simulink model "building_PHPP_v1"  (R2018b)
settings: Solver=ode23s  StartTime=-building.preruntime+8760*3600  StopTime=building.runtime+8760*3600  EnableMultiTasking=on
StartFcn:
  | tic
StopFcn:
  | toc
values from neighbouring files (symbols this model uses):
  A = 7*10*2    (= 140)    [theta_ground_v1.m]    (also in xlswrite1.m = num2cell(data))
  B = A/(0.5 * P)    (= 8.23529411765)    [theta_ground_v1.m]
  building = obj    [BUILDING.m]    (also in create_building_automatic.m = building.save(); ini_building_automatic.m = building.add_variant_hvac(building.variant_hvac, hvac); load_building_automatic.m = building.save())
  C = zeros(1,length(d)+1)    [CONSTRUCTION.m]    (also in DOOR.m = [0 0 0]; WALL.m = [0 0 0]; WINDOW.m = [0 0 0])
  cp = str2num(value)    [CONSTRUCTION.m]
  p = [timevec_weather weather(:,12)]    [BOUNDARY.m]    (also in WEATHER.m = 0; init_carnotUIBK.m = cell2mat(carnotUIBKpaths(i,2)))
  rho = str2num(value)    [CONSTRUCTION.m]    (also in theta_ground_v1.m = 2000)
undefined symbols (not defined in the file or in its folder): Dd, Dreifach, get_building, Qdot_C, Qdot_C_energy, Qdot_H, Qdot_H_energy, Qdot_I_electricity, Qdot_I_electricity_energy, Qdot_I_light, Qdot_I_light_energy, Qdot_I_person, Qdot_I_person_energy, Qdot_S, Qdot_S_energy, Qdot_T_ground, Qdot_T_ground_energy, Qdot_T_neighbour, Qdot_T_neighbour_energy, Qdot_T_opaque, Qdot_T_opaque_energy, Qdot_T_window, Qdot_T_window_energy, Qdot_V_infiltration, Qdot_V_infiltration_energy, Qdot_V_mech, Qdot_V_mech_energy, Qdot_V_window, Qdot_V_window_energy, Tc, Tr, Ts, Wärmeschutzglas, x_CO2, x_H2O, x_VOC
libraries: carnotUIBK x1874, carnot x5, simulink x3
(part 13 of 34)

== system building_PHPP_v1/BUILDING/ZONE_9 ==
  note: VECTOR theta_out
  note: NUMBEROFWALLSINZONES
  WDB : Inport
  GDB : Inport  Port=2
  NDB : Inport  Port=3
  S_in : Inport  Port=4
  Qdot_in : Inport  Port=5
  control : Inport  Port=6
  Add{,2..4} (4 alike) : Sum  Inputs=5
  Add1 : Sum  Inputs=6
  Mux : Mux  Inputs=10
  gain_1 : Subsystem  Variant=on  mask{zone=z.matrix_gains, gains=b.gains, subgain=1}
      mask init: same as building_PHPP_v1/BUILDING/ZONE_1/gain_1
      mask Display:
      | fprintf('GAINS:\n')
      | fprintf('\n%s', ga.name)
  gain_2 : Subsystem  Variant=on  mask{zone=z.matrix_gains, gains=b.gains, subgain=2}
      mask init: same as building_PHPP_v1/BUILDING/ZONE_1/gain_1
      mask Display:
      | fprintf('GAINS:\n')
      | fprintf('\n%s', ga.name)
  gain_3 : Subsystem  Variant=on  mask{zone=z.matrix_gains, gains=b.gains, subgain=3}
      mask init: same as building_PHPP_v1/BUILDING/ZONE_1/gain_1
      mask Display:
      | fprintf('GAINS:\n')
      | fprintf('\n%s', ga.name)
  gain_4 : Subsystem  Variant=on  mask{zone=z.matrix_gains, gains=b.gains, subgain=4}
      mask init: same as building_PHPP_v1/BUILDING/ZONE_1/gain_1
      mask Display:
      | fprintf('GAINS:\n')
      | fprintf('\n%s', ga.name)
  gain_5 : Subsystem  Variant=on  mask{zone=z.matrix_gains, gains=b.gains, subgain=4}
      mask init: same as building_PHPP_v1/BUILDING/ZONE_1/gain_1
      mask Display:
      | fprintf('GAINS:\n')
      | fprintf('\n%s', ga.name)
  infiltration_1 : Subsystem  Variant=on  mask{zone=z.matrix_wi, window=1}
      mask init: same as building_PHPP_v1/BUILDING/ZONE_1/infiltration_1
      mask Display:
      | fprintf('INFILTRATION:\n')
      | %fprintf('\n%s', const.name)
  infiltration_2 : Subsystem  Variant=on  mask{zone=z.matrix_wi, window=2}
      mask init: same as building_PHPP_v1/BUILDING/ZONE_1/infiltration_1
      mask Display:
      | fprintf('INFILTRATION:\n')
      | %fprintf('\n%s', const.name)
  infiltration_3 : Subsystem  Variant=on  mask{zone=z.matrix_wi, window=3}
      mask init: same as building_PHPP_v1/BUILDING/ZONE_1/infiltration_1
      mask Display:
      | fprintf('INFILTRATION:\n')
      | %fprintf('\n%s', const.name)
  infiltration_4 : Subsystem  Variant=on  mask{zone=z.matrix_wi, window=4}
      mask init: same as building_PHPP_v1/BUILDING/ZONE_1/infiltration_1
      mask Display:
      | fprintf('INFILTRATION:\n')
      | %fprintf('\n%s', const.name)
  infiltration_5 : Subsystem  Variant=on  mask{zone=z.matrix_wi, window=5}
      mask init: same as building_PHPP_v1/BUILDING/ZONE_1/infiltration_1
      mask Display:
      | fprintf('INFILTRATION:\n')
      | %fprintf('\n%s', const.name)
  room_node : Subsystem  Variant=on
  wall_1 : Subsystem  Variant=on  mask{zone=z.matrix_wd, construction=b.construction, wall=1}
      mask init: same as building_PHPP_v1/BUILDING/ZONE_1/wall_1
      mask Display:
      | fprintf('CONSTRUCTION:\n')
      | fprintf('\n%s', const.name)
  wall_2 : Subsystem  Variant=on  mask{zone=z.matrix_wd, construction=b.construction, wall=2}
      mask init: same as building_PHPP_v1/BUILDING/ZONE_1/wall_1
      mask Display:
      | fprintf('CONSTRUCTION:\n')
      | fprintf('\n%s', const.name)
  wall_3 : Subsystem  Variant=on  mask{zone=z.matrix_wd, construction=b.construction, wall=3}
      mask init: same as building_PHPP_v1/BUILDING/ZONE_1/wall_1
      mask Display:
      | fprintf('CONSTRUCTION:\n')
      | fprintf('\n%s', const.name)
  wall_4 : Subsystem  Variant=on  mask{zone=z.matrix_wd, construction=b.construction, wall=4}
      mask init: same as building_PHPP_v1/BUILDING/ZONE_1/wall_1
      mask Display:
      | fprintf('CONSTRUCTION:\n')
      | fprintf('\n%s', const.name)
  wall_5 : Subsystem  Variant=on  mask{zone=z.matrix_wd, construction=b.construction, wall=5}
      mask init: same as building_PHPP_v1/BUILDING/ZONE_1/wall_1
      mask Display:
      | fprintf('CONSTRUCTION:\n')
      | fprintf('\n%s', const.name)
  wall_6 : Subsystem  Variant=on  mask{zone=z.matrix_wd, construction=b.construction, wall=6}
      mask init: same as building_PHPP_v1/BUILDING/ZONE_1/wall_1
      mask Display:
      | fprintf('CONSTRUCTION:\n')
      | fprintf('\n%s', const.name)
  window_1 : Subsystem  Variant=on  mask{zone=z.matrix_wi, construction=b.construction, window=1}
      mask init: same as building_PHPP_v1/BUILDING/ZONE_1/window_1
      mask Display:
      | fprintf('CONSTRUCTION:\n')
      | fprintf('\n%s', const.name)
  window_2 : Subsystem  Variant=on  mask{zone=z.matrix_wi, construction=b.construction, window=2}
      mask init: same as building_PHPP_v1/BUILDING/ZONE_1/window_1
      mask Display:
      | fprintf('CONSTRUCTION:\n')
      | fprintf('\n%s', const.name)
  window_3 : Subsystem  Variant=on  mask{zone=z.matrix_wi, construction=b.construction, window=3}
      mask init: same as building_PHPP_v1/BUILDING/ZONE_1/window_1
      mask Display:
      | fprintf('CONSTRUCTION:\n')
      | fprintf('\n%s', const.name)
  window_4 : Subsystem  Variant=on  mask{zone=z.matrix_wi, construction=b.construction, window=4}
      mask init: same as building_PHPP_v1/BUILDING/ZONE_1/window_1
      mask Display:
      | fprintf('CONSTRUCTION:\n')
      | fprintf('\n%s', const.name)
  window_5 : Subsystem  Variant=on  mask{zone=z.matrix_wi, construction=b.construction, window=5}
      mask init: same as building_PHPP_v1/BUILDING/ZONE_1/window_1
      mask Display:
      | fprintf('CONSTRUCTION:\n')
      | fprintf('\n%s', const.name)
  BDB : Outport
  AIB : Outport  Port=2
  theta_out : Outport  Port=3
  wires:
  WDB/1 -> wall_3/1(WDB), wall_4/1(WDB), wall_5/1(WDB), wall_6/1(WDB), window_1/1(WDB), window_4/1(WDB), infiltration_2/2(WDB), infiltration_3/2(WDB), infiltration_4/2(WDB), infiltration_5/2(WDB), infiltration_1/2(WDB), window_5/1(WDB), window_3/1(WDB), window_2/1(WDB), wall_2/1(WDB), wall_1/1(WDB)
  room_node/1(BDB) -> BDB/1
  S_in/1 -> Add/1
  Qdot_in/1 -> wall_1/5(Qdot_in), wall_3/5(Qdot_in), wall_4/5(Qdot_in), wall_6/5(Qdot_in), wall_5/5(Qdot_in), wall_2/5(Qdot_in)
  Add/1 -> room_node/1(sum([S]))
  room_node/3(Qdot_sol) -> wall_3/6(Qdot_sol), wall_4/6(Qdot_sol), wall_6/6(Qdot_sol), wall_5/6(Qdot_sol), wall_2/6(Qdot_sol), wall_1/6(Qdot_sol)
  wall_1/2(theta_out) -> [theta_out_1]
  control/1 -> gain_2/2(control), gain_3/2(control), infiltration_1/3(control), infiltration_2/3(control), infiltration_3/3(control), infiltration_4/3(control), infiltration_5/3(control), gain_5/2(control), gain_4/2(control), gain_1/2(control), window_5/3(control), window_4/3(control), window_3/3(control), window_2/3(control), window_1/3(control)
  room_node/2(AIB) -> AIB/1, wall_3/4(AIB), wall_4/4(AIB), wall_5/4(AIB), wall_6/4(AIB), gain_2/1(AIB), gain_3/1(AIB), infiltration_2/1(AIB), infiltration_3/1(AIB), infiltration_4/1(AIB), infiltration_5/1(AIB), infiltration_1/1(AIB), gain_5/1(AIB), gain_4/1(AIB), gain_1/1(AIB), window_5/2(AIB), window_4/2(AIB), window_3/2(AIB), window_2/2(AIB), window_1/2(AIB), wall_2/4(AIB), wall_1/4(AIB)
  Mux/1 -> theta_out/1
  [theta_out_1] -> Mux/1
  [theta_out_2] -> Mux/2
  [theta_out_10] -> Mux/10
  [theta_out_9] -> Mux/9
  [theta_out_8] -> Mux/8
  [theta_out_7] -> Mux/7
  [theta_out_6] -> Mux/6
  [theta_out_5] -> Mux/5
  [theta_out_4] -> Mux/4
  [theta_out_3] -> Mux/3
  wall_2/2(theta_out) -> [theta_out_2]
  GDB/1 -> wall_1/2(GDB), wall_3/2(GDB), wall_4/2(GDB), wall_6/2(GDB), wall_5/2(GDB), wall_2/2(GDB)
  wall_3/2(theta_out) -> [theta_out_3]
  wall_4/2(theta_out) -> [theta_out_4]
  wall_5/2(theta_out) -> [theta_out_5]
  wall_6/2(theta_out) -> [theta_out_6]
  NDB/1 -> wall_1/3(NDB), wall_3/3(NDB), wall_4/3(NDB), wall_6/3(NDB), wall_5/3(NDB), wall_2/3(NDB)
  wall_1/1("[S]") -> Add1/1
  wall_6/1("[S]") -> Add1/6
  wall_2/1("[S]") -> Add1/2
  wall_3/1("[S]") -> Add1/3
  wall_4/1("[S]") -> Add1/4
  wall_5/1("[S]") -> Add1/5
  Add1/1 -> Add/2
  window_1/1("[S]") -> Add2/1
  window_5/1("[S]") -> Add2/5
  window_2/1("[S]") -> Add2/2
  window_3/1("[S]") -> Add2/3
  window_4/1("[S]") -> Add2/4
  Add2/1 -> Add/3
  gain_1/1("[S]") -> Add3/1
  gain_5/1("[S]") -> Add3/5
  gain_2/1("[S]") -> Add3/2
  gain_3/1("[S]") -> Add3/3
  gain_4/1("[S]") -> Add3/4
  Add3/1 -> Add/4
  infiltration_1/1("[S]") -> Add4/1
  infiltration_5/1("[S]") -> Add4/5
  infiltration_4/1("[S]") -> Add4/4
  infiltration_3/1("[S]") -> Add4/3
  infiltration_2/1("[S]") -> Add4/2
  Add4/1 -> Add/5

== system building_PHPP_v1/DATALOGGER/AIBz1 ==
  AIB : Inport
  AIB_initialize : carnotUIBK/room_node/EMPTY/AIB_initialize  SystemSampleTime=-1
  Bus Assignment1 : BusAssignment  AssignedSignals=Ts,Tc,Tr,x_H2O,x_CO2,x_VOC,rho,cp,p
  Bus Selector1 : BusSelector  OutputSignals=Ts,Tc,Tr,x_H2O,x_CO2,x_VOC,rho,cp,p
  AIB' : Outport
  wires:
  Bus Assignment1/1 -> AIB'/1
  AIB/1 -> Bus Selector1/1
  AIB_initialize/1 -> Bus Assignment1/1
  Bus Selector1/1 -> Bus Assignment1/2  "<Ts>"
  Bus Selector1/3 -> Bus Assignment1/4  "<Tr>"
  Bus Selector1/9 -> Bus Assignment1/10  "<p>"
  Bus Selector1/4 -> Bus Assignment1/5  "<x_H2O>"
  Bus Selector1/2 -> Bus Assignment1/3  "<Tc>"
  Bus Selector1/5 -> Bus Assignment1/6  "<x_CO2>"
  Bus Selector1/6 -> Bus Assignment1/7  "<x_VOC>"
  Bus Selector1/7 -> Bus Assignment1/8  "<rho>"
  Bus Selector1/8 -> Bus Assignment1/9  "<cp>"

== system building_PHPP_v1/DATALOGGER/AIBz10 ==
  AIB : Inport
  AIB_initialize : carnotUIBK/room_node/EMPTY/AIB_initialize  SystemSampleTime=-1
  Bus Assignment1 : BusAssignment  AssignedSignals=Ts,Tc,Tr,x_H2O,x_CO2,x_VOC,rho,cp,p
  Bus Selector1 : BusSelector  OutputSignals=Ts,Tc,Tr,x_H2O,x_CO2,x_VOC,rho,cp,p
  AIB' : Outport
  wires:
  Bus Selector1/8 -> Bus Assignment1/9  "<cp>"
  Bus Selector1/7 -> Bus Assignment1/8  "<rho>"
  Bus Selector1/6 -> Bus Assignment1/7  "<x_VOC>"
  Bus Selector1/5 -> Bus Assignment1/6  "<x_CO2>"
  Bus Selector1/2 -> Bus Assignment1/3  "<Tc>"
  Bus Selector1/4 -> Bus Assignment1/5  "<x_H2O>"
  Bus Selector1/9 -> Bus Assignment1/10  "<p>"
  Bus Selector1/3 -> Bus Assignment1/4  "<Tr>"
  Bus Selector1/1 -> Bus Assignment1/2  "<Ts>"
  AIB_initialize/1 -> Bus Assignment1/1
  AIB/1 -> Bus Selector1/1
  Bus Assignment1/1 -> AIB'/1

== system building_PHPP_v1/DATALOGGER/AIBz2 ==
  AIB : Inport
  AIB_initialize : carnotUIBK/room_node/EMPTY/AIB_initialize  SystemSampleTime=-1
  Bus Assignment1 : BusAssignment  AssignedSignals=Ts,Tc,Tr,x_H2O,x_CO2,x_VOC,rho,cp,p
  Bus Selector1 : BusSelector  OutputSignals=Ts,Tc,Tr,x_H2O,x_CO2,x_VOC,rho,cp,p
  AIB' : Outport
  wires:
  Bus Selector1/8 -> Bus Assignment1/9  "<cp>"
  Bus Selector1/7 -> Bus Assignment1/8  "<rho>"
  Bus Selector1/6 -> Bus Assignment1/7  "<x_VOC>"
  Bus Selector1/5 -> Bus Assignment1/6  "<x_CO2>"
  Bus Selector1/2 -> Bus Assignment1/3  "<Tc>"
  Bus Selector1/4 -> Bus Assignment1/5  "<x_H2O>"
  Bus Selector1/9 -> Bus Assignment1/10  "<p>"
  Bus Selector1/3 -> Bus Assignment1/4  "<Tr>"
  Bus Selector1/1 -> Bus Assignment1/2  "<Ts>"
  AIB_initialize/1 -> Bus Assignment1/1
  AIB/1 -> Bus Selector1/1
  Bus Assignment1/1 -> AIB'/1

== system building_PHPP_v1/DATALOGGER/AIBz3 ==
  AIB : Inport
  AIB_initialize : carnotUIBK/room_node/EMPTY/AIB_initialize  SystemSampleTime=-1
  Bus Assignment1 : BusAssignment  AssignedSignals=Ts,Tc,Tr,x_H2O,x_CO2,x_VOC,rho,cp,p
  Bus Selector1 : BusSelector  OutputSignals=Ts,Tc,Tr,x_H2O,x_CO2,x_VOC,rho,cp,p
  AIB' : Outport
  wires:
  Bus Assignment1/1 -> AIB'/1
  AIB/1 -> Bus Selector1/1
  AIB_initialize/1 -> Bus Assignment1/1
  Bus Selector1/1 -> Bus Assignment1/2  "<Ts>"
  Bus Selector1/3 -> Bus Assignment1/4  "<Tr>"
  Bus Selector1/9 -> Bus Assignment1/10  "<p>"
  Bus Selector1/4 -> Bus Assignment1/5  "<x_H2O>"
  Bus Selector1/2 -> Bus Assignment1/3  "<Tc>"
  Bus Selector1/5 -> Bus Assignment1/6  "<x_CO2>"
  Bus Selector1/6 -> Bus Assignment1/7  "<x_VOC>"
  Bus Selector1/7 -> Bus Assignment1/8  "<rho>"
  Bus Selector1/8 -> Bus Assignment1/9  "<cp>"

== system building_PHPP_v1/DATALOGGER/AIBz4 ==
  AIB : Inport
  AIB_initialize : carnotUIBK/room_node/EMPTY/AIB_initialize  SystemSampleTime=-1
  Bus Assignment1 : BusAssignment  AssignedSignals=Ts,Tc,Tr,x_H2O,x_CO2,x_VOC,rho,cp,p
  Bus Selector1 : BusSelector  OutputSignals=Ts,Tc,Tr,x_H2O,x_CO2,x_VOC,rho,cp,p
  AIB' : Outport
  wires:
  Bus Selector1/8 -> Bus Assignment1/9  "<cp>"
  Bus Selector1/7 -> Bus Assignment1/8  "<rho>"
  Bus Selector1/6 -> Bus Assignment1/7  "<x_VOC>"
  Bus Selector1/5 -> Bus Assignment1/6  "<x_CO2>"
  Bus Selector1/2 -> Bus Assignment1/3  "<Tc>"
  Bus Selector1/4 -> Bus Assignment1/5  "<x_H2O>"
  Bus Selector1/9 -> Bus Assignment1/10  "<p>"
  Bus Selector1/3 -> Bus Assignment1/4  "<Tr>"
  Bus Selector1/1 -> Bus Assignment1/2  "<Ts>"
  AIB_initialize/1 -> Bus Assignment1/1
  AIB/1 -> Bus Selector1/1
  Bus Assignment1/1 -> AIB'/1

== system building_PHPP_v1/DATALOGGER/AIBz5 ==
  AIB : Inport
  AIB_initialize : carnotUIBK/room_node/EMPTY/AIB_initialize  SystemSampleTime=-1
  Bus Assignment1 : BusAssignment  AssignedSignals=Ts,Tc,Tr,x_H2O,x_CO2,x_VOC,rho,cp,p
  Bus Selector1 : BusSelector  OutputSignals=Ts,Tc,Tr,x_H2O,x_CO2,x_VOC,rho,cp,p
  AIB' : Outport
  wires:
  Bus Assignment1/1 -> AIB'/1
  AIB/1 -> Bus Selector1/1
  AIB_initialize/1 -> Bus Assignment1/1
  Bus Selector1/1 -> Bus Assignment1/2  "<Ts>"
  Bus Selector1/3 -> Bus Assignment1/4  "<Tr>"
  Bus Selector1/9 -> Bus Assignment1/10  "<p>"
  Bus Selector1/4 -> Bus Assignment1/5  "<x_H2O>"
  Bus Selector1/2 -> Bus Assignment1/3  "<Tc>"
  Bus Selector1/5 -> Bus Assignment1/6  "<x_CO2>"
  Bus Selector1/6 -> Bus Assignment1/7  "<x_VOC>"
  Bus Selector1/7 -> Bus Assignment1/8  "<rho>"
  Bus Selector1/8 -> Bus Assignment1/9  "<cp>"

== system building_PHPP_v1/DATALOGGER/AIBz6 ==
  AIB : Inport
  AIB_initialize : carnotUIBK/room_node/EMPTY/AIB_initialize  SystemSampleTime=-1
  Bus Assignment1 : BusAssignment  AssignedSignals=Ts,Tc,Tr,x_H2O,x_CO2,x_VOC,rho,cp,p
  Bus Selector1 : BusSelector  OutputSignals=Ts,Tc,Tr,x_H2O,x_CO2,x_VOC,rho,cp,p
  AIB' : Outport
  wires:
  Bus Selector1/8 -> Bus Assignment1/9  "<cp>"
  Bus Selector1/7 -> Bus Assignment1/8  "<rho>"
  Bus Selector1/6 -> Bus Assignment1/7  "<x_VOC>"
  Bus Selector1/5 -> Bus Assignment1/6  "<x_CO2>"
  Bus Selector1/2 -> Bus Assignment1/3  "<Tc>"
  Bus Selector1/4 -> Bus Assignment1/5  "<x_H2O>"
  Bus Selector1/9 -> Bus Assignment1/10  "<p>"
  Bus Selector1/3 -> Bus Assignment1/4  "<Tr>"
  Bus Selector1/1 -> Bus Assignment1/2  "<Ts>"
  AIB_initialize/1 -> Bus Assignment1/1
  AIB/1 -> Bus Selector1/1
  Bus Assignment1/1 -> AIB'/1

== system building_PHPP_v1/DATALOGGER/AIBz7 ==
  AIB : Inport
  AIB_initialize : carnotUIBK/room_node/EMPTY/AIB_initialize  SystemSampleTime=-1
  Bus Assignment1 : BusAssignment  AssignedSignals=Ts,Tc,Tr,x_H2O,x_CO2,x_VOC,rho,cp,p
  Bus Selector1 : BusSelector  OutputSignals=Ts,Tc,Tr,x_H2O,x_CO2,x_VOC,rho,cp,p
  AIB' : Outport
  wires:
  Bus Assignment1/1 -> AIB'/1
  AIB/1 -> Bus Selector1/1
  AIB_initialize/1 -> Bus Assignment1/1
  Bus Selector1/1 -> Bus Assignment1/2  "<Ts>"
  Bus Selector1/3 -> Bus Assignment1/4  "<Tr>"
  Bus Selector1/9 -> Bus Assignment1/10  "<p>"
  Bus Selector1/4 -> Bus Assignment1/5  "<x_H2O>"
  Bus Selector1/2 -> Bus Assignment1/3  "<Tc>"
  Bus Selector1/5 -> Bus Assignment1/6  "<x_CO2>"
  Bus Selector1/6 -> Bus Assignment1/7  "<x_VOC>"
  Bus Selector1/7 -> Bus Assignment1/8  "<rho>"
  Bus Selector1/8 -> Bus Assignment1/9  "<cp>"

== system building_PHPP_v1/DATALOGGER/AIBz8 ==
  AIB : Inport
  AIB_initialize : carnotUIBK/room_node/EMPTY/AIB_initialize  SystemSampleTime=-1
  Bus Assignment1 : BusAssignment  AssignedSignals=Ts,Tc,Tr,x_H2O,x_CO2,x_VOC,rho,cp,p
  Bus Selector1 : BusSelector  OutputSignals=Ts,Tc,Tr,x_H2O,x_CO2,x_VOC,rho,cp,p
  AIB' : Outport
  wires:
  Bus Selector1/8 -> Bus Assignment1/9  "<cp>"
  Bus Selector1/7 -> Bus Assignment1/8  "<rho>"
  Bus Selector1/6 -> Bus Assignment1/7  "<x_VOC>"
  Bus Selector1/5 -> Bus Assignment1/6  "<x_CO2>"
  Bus Selector1/2 -> Bus Assignment1/3  "<Tc>"
  Bus Selector1/4 -> Bus Assignment1/5  "<x_H2O>"
  Bus Selector1/9 -> Bus Assignment1/10  "<p>"
  Bus Selector1/3 -> Bus Assignment1/4  "<Tr>"
  Bus Selector1/1 -> Bus Assignment1/2  "<Ts>"
  AIB_initialize/1 -> Bus Assignment1/1
  AIB/1 -> Bus Selector1/1
  Bus Assignment1/1 -> AIB'/1

== system building_PHPP_v1/DATALOGGER/AIBz9 ==
  AIB : Inport
  AIB_initialize : carnotUIBK/room_node/EMPTY/AIB_initialize  SystemSampleTime=-1
  Bus Assignment1 : BusAssignment  AssignedSignals=Ts,Tc,Tr,x_H2O,x_CO2,x_VOC,rho,cp,p
  Bus Selector1 : BusSelector  OutputSignals=Ts,Tc,Tr,x_H2O,x_CO2,x_VOC,rho,cp,p
  AIB' : Outport
  wires:
  Bus Assignment1/1 -> AIB'/1
  AIB/1 -> Bus Selector1/1
  AIB_initialize/1 -> Bus Assignment1/1
  Bus Selector1/1 -> Bus Assignment1/2  "<Ts>"
  Bus Selector1/3 -> Bus Assignment1/4  "<Tr>"
  Bus Selector1/9 -> Bus Assignment1/10  "<p>"
  Bus Selector1/4 -> Bus Assignment1/5  "<x_H2O>"
  Bus Selector1/2 -> Bus Assignment1/3  "<Tc>"
  Bus Selector1/5 -> Bus Assignment1/6  "<x_CO2>"
  Bus Selector1/6 -> Bus Assignment1/7  "<x_VOC>"
  Bus Selector1/7 -> Bus Assignment1/8  "<rho>"
  Bus Selector1/8 -> Bus Assignment1/9  "<cp>"

== system building_PHPP_v1/DATALOGGER/logger_AIB ==
  AIB : Inport
  Enable : EnablePort
  saveAIB : ToWorkspace  VariableName=saveAIB  SaveFormat=Timeseries  SampleTime=building.get_building().sampletime_1
  wires:
  AIB/1 -> saveAIB/1

== system building_PHPP_v1/DATALOGGER/logger_BDB ==
  note: CHANGE BDB TO THE CORRESPONDING ZONE!!!!
  BDB : Inport
  Enable : EnablePort
  Bus Creator : BusCreator  Inputs=2
  Bus Creator1 : BusCreator  Inputs=10
  saveBDB : ToWorkspace  VariableName=saveBDB  SaveFormat=Timeseries  SampleTime=building.get_building().sampletime_1
  z1 : Subsystem
  z10 : Subsystem
  z2 : Subsystem
  z3 : Subsystem
  z4 : Subsystem
  z5 : Subsystem
  z6 : Subsystem
  z7 : Subsystem
  z8 : Subsystem
  z9 : Subsystem
  wires:
  BDB/1 -> Bus Creator/1, z1/1(BDB), z2/1(BDB), z3/1(BDB), z4/1(BDB), z5/1(BDB), z6/1(BDB), z7/1(BDB), z8/1(BDB), z10/1(BDB), z9/1(BDB)  "power"
  Bus Creator/1 -> saveBDB/1
  z1/1(BDBenergy) -> Bus Creator1/1  "z1"
  z4/1(BDBenergy) -> Bus Creator1/4  "z4"
  z3/1(BDBenergy) -> Bus Creator1/3  "z3"
  z2/1(BDBenergy) -> Bus Creator1/2  "z2"
  z10/1(BDBenergy) -> Bus Creator1/10  "z10"
  z9/1(BDBenergy) -> Bus Creator1/9  "z9"
  z8/1(BDBenergy) -> Bus Creator1/8  "z8"
  z7/1(BDBenergy) -> Bus Creator1/7  "z7"
  z6/1(BDBenergy) -> Bus Creator1/6  "z6"
  z5/1(BDBenergy) -> Bus Creator1/5  "z5"
  Bus Creator1/1 -> Bus Creator/2  "energy"

== system building_PHPP_v1/DATALOGGER/logger_BOUNDARY ==
  BOUNDARY : Inport
  Enable : EnablePort
  Bus Creator : BusCreator  Inputs=2
  Bus Creator1 : BusCreator  Inputs=4
  Bus Selector : BusSelector  OutputSignals=WDB.Solar_Radiation_beam_normal,WDB.Solar_Radiation_diffuse_horizontal,WDB.Solar_Radiation_direct_surface,WDB.Solar_Radiation_diffuse_surface  OutputAsBus=on
  Demux : Demux
  Integrator : Integrator
  Ws->kWh : Gain  Gain=1/3600/1000
  saveBOUNDARY : ToWorkspace  VariableName=saveBOUNDARY  SaveFormat=Timeseries  SampleTime=building.get_building().sampletime_1
  wires:
  BOUNDARY/1 -> Bus Selector/1, Bus Creator/1  "power"
  Bus Creator/1 -> saveBOUNDARY/1
  Bus Selector/1 -> Integrator/1
  Integrator/1 -> Ws->kWh/1
  Demux/1 -> Bus Creator1/1  "Solar_Radiation_beam_normal_Energy"
  Demux/2 -> Bus Creator1/2  "Solar_Radiation_diffuse_horizontal_Energy"
  Demux/4 -> Bus Creator1/4  "Solar_Radiation_diffuse_surface_Energy"
  Demux/3 -> Bus Creator1/3  "Solar_Radiation_direct_surface_Energy"
  Bus Creator1/1 -> Bus Creator/2  "energy"
  Ws->kWh/1 -> Demux/1

== system building_PHPP_v1/DATALOGGER/logger_HVAC ==
  HVAC : Inport
  Enable : EnablePort
  saveHVAC : ToWorkspace  VariableName=saveHVAC  SaveFormat=Timeseries  SampleTime=building.get_building().sampletime_1
  wires:
  HVAC/1 -> saveHVAC/1

== system building_PHPP_v1/DATALOGGER/z1 ==
  BDB : Inport
  BDB_initialize : carnotUIBK/room_node/EMPTY/BDB_initialize  SystemSampleTime=-1
  Bus Assignment : BusAssignment  AssignedSignals=Qdot_T_opaque,Qdot_T_ground,Qdot_T_neighbour,Qdot_T_window,Qdot_V_mech,Qdot_V_window,Qdot_V_infiltration,Qdot_S,Qdot_I_person,Qdot_I_light,Qdot_I_electricity,Qdot_H,Qdot_C
  Bus Selector1 : BusSelector  OutputSignals=Qdot_T_opaque,Qdot_T_ground,Qdot_T_neighbour,Qdot_T_window,Qdot_V_mech,Qdot_V_window,Qdot_V_infiltration,Qdot_S,Qdot_I_person,Qdot_I_light,Qdot_I_electricity,Qdot_H,Qdot_C
  BDB' : Outport
  wires:
  BDB/1 -> Bus Selector1/1
  Bus Assignment/1 -> BDB'/1
  BDB_initialize/1 -> Bus Assignment/1
  Bus Selector1/1 -> Bus Assignment/2  "<Qdot_T_opaque>"
  Bus Selector1/13 -> Bus Assignment/14  "<Qdot_C>"
  Bus Selector1/12 -> Bus Assignment/13  "<Qdot_H>"
  Bus Selector1/11 -> Bus Assignment/12  "<Qdot_I_electricity>"
  Bus Selector1/10 -> Bus Assignment/11  "<Qdot_I_light>"
  Bus Selector1/9 -> Bus Assignment/10  "<Qdot_I_person>"
  Bus Selector1/8 -> Bus Assignment/9  "<Qdot_S>"
  Bus Selector1/7 -> Bus Assignment/8  "<Qdot_V_infiltration>"
  Bus Selector1/6 -> Bus Assignment/7  "<Qdot_V_window>"
  Bus Selector1/5 -> Bus Assignment/6  "<Qdot_V_mech>"
  Bus Selector1/4 -> Bus Assignment/5  "<Qdot_T_window>"
  Bus Selector1/3 -> Bus Assignment/4  "<Qdot_T_neighbour>"
  Bus Selector1/2 -> Bus Assignment/3  "<Qdot_T_ground>"

== system building_PHPP_v1/DATALOGGER/z10 ==
  BDB : Inport
  BDB_initialize : carnotUIBK/room_node/EMPTY/BDB_initialize  SystemSampleTime=-1
  Bus Assignment : BusAssignment  AssignedSignals=Qdot_T_opaque,Qdot_T_ground,Qdot_T_neighbour,Qdot_T_window,Qdot_V_mech,Qdot_V_window,Qdot_V_infiltration,Qdot_S,Qdot_I_person,Qdot_I_light,Qdot_I_electricity,Qdot_H,Qdot_C
  Bus Selector1 : BusSelector  OutputSignals=Qdot_T_opaque,Qdot_T_ground,Qdot_T_neighbour,Qdot_T_window,Qdot_V_mech,Qdot_V_window,Qdot_V_infiltration,Qdot_S,Qdot_I_person,Qdot_I_light,Qdot_I_electricity,Qdot_H,Qdot_C
  BDB' : Outport
  wires:
  Bus Selector1/2 -> Bus Assignment/3  "<Qdot_T_ground>"
  Bus Selector1/3 -> Bus Assignment/4  "<Qdot_T_neighbour>"
  Bus Selector1/4 -> Bus Assignment/5  "<Qdot_T_window>"
  Bus Selector1/5 -> Bus Assignment/6  "<Qdot_V_mech>"
  Bus Selector1/6 -> Bus Assignment/7  "<Qdot_V_window>"
  Bus Selector1/7 -> Bus Assignment/8  "<Qdot_V_infiltration>"
  Bus Selector1/8 -> Bus Assignment/9  "<Qdot_S>"
  Bus Selector1/9 -> Bus Assignment/10  "<Qdot_I_person>"
  Bus Selector1/10 -> Bus Assignment/11  "<Qdot_I_light>"
  Bus Selector1/11 -> Bus Assignment/12  "<Qdot_I_electricity>"
  Bus Selector1/12 -> Bus Assignment/13  "<Qdot_H>"
  Bus Selector1/13 -> Bus Assignment/14  "<Qdot_C>"
  Bus Selector1/1 -> Bus Assignment/2  "<Qdot_T_opaque>"
  BDB_initialize/1 -> Bus Assignment/1
  Bus Assignment/1 -> BDB'/1
  BDB/1 -> Bus Selector1/1

== system building_PHPP_v1/DATALOGGER/z2 ==
  BDB : Inport
  BDB_initialize : carnotUIBK/room_node/EMPTY/BDB_initialize  SystemSampleTime=-1
  Bus Assignment : BusAssignment  AssignedSignals=Qdot_T_opaque,Qdot_T_ground,Qdot_T_neighbour,Qdot_T_window,Qdot_V_mech,Qdot_V_window,Qdot_V_infiltration,Qdot_S,Qdot_I_person,Qdot_I_light,Qdot_I_electricity,Qdot_H,Qdot_C
  Bus Selector1 : BusSelector  OutputSignals=Qdot_T_opaque,Qdot_T_ground,Qdot_T_neighbour,Qdot_T_window,Qdot_V_mech,Qdot_V_window,Qdot_V_infiltration,Qdot_S,Qdot_I_person,Qdot_I_light,Qdot_I_electricity,Qdot_H,Qdot_C
  BDB' : Outport
  wires:
  Bus Selector1/2 -> Bus Assignment/3  "<Qdot_T_ground>"
  Bus Selector1/3 -> Bus Assignment/4  "<Qdot_T_neighbour>"
  Bus Selector1/4 -> Bus Assignment/5  "<Qdot_T_window>"
  Bus Selector1/5 -> Bus Assignment/6  "<Qdot_V_mech>"
  Bus Selector1/6 -> Bus Assignment/7  "<Qdot_V_window>"
  Bus Selector1/7 -> Bus Assignment/8  "<Qdot_V_infiltration>"
  Bus Selector1/8 -> Bus Assignment/9  "<Qdot_S>"
  Bus Selector1/9 -> Bus Assignment/10  "<Qdot_I_person>"
  Bus Selector1/10 -> Bus Assignment/11  "<Qdot_I_light>"
  Bus Selector1/11 -> Bus Assignment/12  "<Qdot_I_electricity>"
  Bus Selector1/12 -> Bus Assignment/13  "<Qdot_H>"
  Bus Selector1/13 -> Bus Assignment/14  "<Qdot_C>"
  Bus Selector1/1 -> Bus Assignment/2  "<Qdot_T_opaque>"
  BDB_initialize/1 -> Bus Assignment/1
  Bus Assignment/1 -> BDB'/1
  BDB/1 -> Bus Selector1/1

== system building_PHPP_v1/DATALOGGER/z3 ==
  BDB : Inport
  BDB_initialize : carnotUIBK/room_node/EMPTY/BDB_initialize  SystemSampleTime=-1
  Bus Assignment : BusAssignment  AssignedSignals=Qdot_T_opaque,Qdot_T_ground,Qdot_T_neighbour,Qdot_T_window,Qdot_V_mech,Qdot_V_window,Qdot_V_infiltration,Qdot_S,Qdot_I_person,Qdot_I_light,Qdot_I_electricity,Qdot_H,Qdot_C
  Bus Selector1 : BusSelector  OutputSignals=Qdot_T_opaque,Qdot_T_ground,Qdot_T_neighbour,Qdot_T_window,Qdot_V_mech,Qdot_V_window,Qdot_V_infiltration,Qdot_S,Qdot_I_person,Qdot_I_light,Qdot_I_electricity,Qdot_H,Qdot_C
  BDB' : Outport
  wires:
  BDB/1 -> Bus Selector1/1
  Bus Assignment/1 -> BDB'/1
  BDB_initialize/1 -> Bus Assignment/1
  Bus Selector1/1 -> Bus Assignment/2  "<Qdot_T_opaque>"
  Bus Selector1/13 -> Bus Assignment/14  "<Qdot_C>"
  Bus Selector1/12 -> Bus Assignment/13  "<Qdot_H>"
  Bus Selector1/11 -> Bus Assignment/12  "<Qdot_I_electricity>"
  Bus Selector1/10 -> Bus Assignment/11  "<Qdot_I_light>"
  Bus Selector1/9 -> Bus Assignment/10  "<Qdot_I_person>"
  Bus Selector1/8 -> Bus Assignment/9  "<Qdot_S>"
  Bus Selector1/7 -> Bus Assignment/8  "<Qdot_V_infiltration>"
  Bus Selector1/6 -> Bus Assignment/7  "<Qdot_V_window>"
  Bus Selector1/5 -> Bus Assignment/6  "<Qdot_V_mech>"
  Bus Selector1/4 -> Bus Assignment/5  "<Qdot_T_window>"
  Bus Selector1/3 -> Bus Assignment/4  "<Qdot_T_neighbour>"
  Bus Selector1/2 -> Bus Assignment/3  "<Qdot_T_ground>"

== system building_PHPP_v1/DATALOGGER/z4 ==
  BDB : Inport
  BDB_initialize : carnotUIBK/room_node/EMPTY/BDB_initialize  SystemSampleTime=-1
  Bus Assignment : BusAssignment  AssignedSignals=Qdot_T_opaque,Qdot_T_ground,Qdot_T_neighbour,Qdot_T_window,Qdot_V_mech,Qdot_V_window,Qdot_V_infiltration,Qdot_S,Qdot_I_person,Qdot_I_light,Qdot_I_electricity,Qdot_H,Qdot_C
  Bus Selector1 : BusSelector  OutputSignals=Qdot_T_opaque,Qdot_T_ground,Qdot_T_neighbour,Qdot_T_window,Qdot_V_mech,Qdot_V_window,Qdot_V_infiltration,Qdot_S,Qdot_I_person,Qdot_I_light,Qdot_I_electricity,Qdot_H,Qdot_C
  BDB' : Outport
  wires:
  Bus Selector1/2 -> Bus Assignment/3  "<Qdot_T_ground>"
  Bus Selector1/3 -> Bus Assignment/4  "<Qdot_T_neighbour>"
  Bus Selector1/4 -> Bus Assignment/5  "<Qdot_T_window>"
  Bus Selector1/5 -> Bus Assignment/6  "<Qdot_V_mech>"
  Bus Selector1/6 -> Bus Assignment/7  "<Qdot_V_window>"
  Bus Selector1/7 -> Bus Assignment/8  "<Qdot_V_infiltration>"
  Bus Selector1/8 -> Bus Assignment/9  "<Qdot_S>"
  Bus Selector1/9 -> Bus Assignment/10  "<Qdot_I_person>"
  Bus Selector1/10 -> Bus Assignment/11  "<Qdot_I_light>"
  Bus Selector1/11 -> Bus Assignment/12  "<Qdot_I_electricity>"
  Bus Selector1/12 -> Bus Assignment/13  "<Qdot_H>"
  Bus Selector1/13 -> Bus Assignment/14  "<Qdot_C>"
  Bus Selector1/1 -> Bus Assignment/2  "<Qdot_T_opaque>"
  BDB_initialize/1 -> Bus Assignment/1
  Bus Assignment/1 -> BDB'/1
  BDB/1 -> Bus Selector1/1

== system building_PHPP_v1/DATALOGGER/z5 ==
  BDB : Inport
  BDB_initialize : carnotUIBK/room_node/EMPTY/BDB_initialize  SystemSampleTime=-1
  Bus Assignment : BusAssignment  AssignedSignals=Qdot_T_opaque,Qdot_T_ground,Qdot_T_neighbour,Qdot_T_window,Qdot_V_mech,Qdot_V_window,Qdot_V_infiltration,Qdot_S,Qdot_I_person,Qdot_I_light,Qdot_I_electricity,Qdot_H,Qdot_C
  Bus Selector1 : BusSelector  OutputSignals=Qdot_T_opaque,Qdot_T_ground,Qdot_T_neighbour,Qdot_T_window,Qdot_V_mech,Qdot_V_window,Qdot_V_infiltration,Qdot_S,Qdot_I_person,Qdot_I_light,Qdot_I_electricity,Qdot_H,Qdot_C
  BDB' : Outport
  wires:
  BDB/1 -> Bus Selector1/1
  Bus Assignment/1 -> BDB'/1
  BDB_initialize/1 -> Bus Assignment/1
  Bus Selector1/1 -> Bus Assignment/2  "<Qdot_T_opaque>"
  Bus Selector1/13 -> Bus Assignment/14  "<Qdot_C>"
  Bus Selector1/12 -> Bus Assignment/13  "<Qdot_H>"
  Bus Selector1/11 -> Bus Assignment/12  "<Qdot_I_electricity>"
  Bus Selector1/10 -> Bus Assignment/11  "<Qdot_I_light>"
  Bus Selector1/9 -> Bus Assignment/10  "<Qdot_I_person>"
  Bus Selector1/8 -> Bus Assignment/9  "<Qdot_S>"
  Bus Selector1/7 -> Bus Assignment/8  "<Qdot_V_infiltration>"
  Bus Selector1/6 -> Bus Assignment/7  "<Qdot_V_window>"
  Bus Selector1/5 -> Bus Assignment/6  "<Qdot_V_mech>"
  Bus Selector1/4 -> Bus Assignment/5  "<Qdot_T_window>"
  Bus Selector1/3 -> Bus Assignment/4  "<Qdot_T_neighbour>"
  Bus Selector1/2 -> Bus Assignment/3  "<Qdot_T_ground>"

== system building_PHPP_v1/DATALOGGER/z6 ==
  BDB : Inport
  BDB_initialize : carnotUIBK/room_node/EMPTY/BDB_initialize  SystemSampleTime=-1
  Bus Assignment : BusAssignment  AssignedSignals=Qdot_T_opaque,Qdot_T_ground,Qdot_T_neighbour,Qdot_T_window,Qdot_V_mech,Qdot_V_window,Qdot_V_infiltration,Qdot_S,Qdot_I_person,Qdot_I_light,Qdot_I_electricity,Qdot_H,Qdot_C
  Bus Selector1 : BusSelector  OutputSignals=Qdot_T_opaque,Qdot_T_ground,Qdot_T_neighbour,Qdot_T_window,Qdot_V_mech,Qdot_V_window,Qdot_V_infiltration,Qdot_S,Qdot_I_person,Qdot_I_light,Qdot_I_electricity,Qdot_H,Qdot_C
  BDB' : Outport
  wires:
  Bus Selector1/2 -> Bus Assignment/3  "<Qdot_T_ground>"
  Bus Selector1/3 -> Bus Assignment/4  "<Qdot_T_neighbour>"
  Bus Selector1/4 -> Bus Assignment/5  "<Qdot_T_window>"
  Bus Selector1/5 -> Bus Assignment/6  "<Qdot_V_mech>"
  Bus Selector1/6 -> Bus Assignment/7  "<Qdot_V_window>"
  Bus Selector1/7 -> Bus Assignment/8  "<Qdot_V_infiltration>"
  Bus Selector1/8 -> Bus Assignment/9  "<Qdot_S>"
  Bus Selector1/9 -> Bus Assignment/10  "<Qdot_I_person>"
  Bus Selector1/10 -> Bus Assignment/11  "<Qdot_I_light>"
  Bus Selector1/11 -> Bus Assignment/12  "<Qdot_I_electricity>"
  Bus Selector1/12 -> Bus Assignment/13  "<Qdot_H>"
  Bus Selector1/13 -> Bus Assignment/14  "<Qdot_C>"
  Bus Selector1/1 -> Bus Assignment/2  "<Qdot_T_opaque>"
  BDB_initialize/1 -> Bus Assignment/1
  Bus Assignment/1 -> BDB'/1
  BDB/1 -> Bus Selector1/1

== system building_PHPP_v1/DATALOGGER/z7 ==
  BDB : Inport
  BDB_initialize : carnotUIBK/room_node/EMPTY/BDB_initialize  SystemSampleTime=-1
  Bus Assignment : BusAssignment  AssignedSignals=Qdot_T_opaque,Qdot_T_ground,Qdot_T_neighbour,Qdot_T_window,Qdot_V_mech,Qdot_V_window,Qdot_V_infiltration,Qdot_S,Qdot_I_person,Qdot_I_light,Qdot_I_electricity,Qdot_H,Qdot_C
  Bus Selector1 : BusSelector  OutputSignals=Qdot_T_opaque,Qdot_T_ground,Qdot_T_neighbour,Qdot_T_window,Qdot_V_mech,Qdot_V_window,Qdot_V_infiltration,Qdot_S,Qdot_I_person,Qdot_I_light,Qdot_I_electricity,Qdot_H,Qdot_C
  BDB' : Outport
  wires:
  BDB/1 -> Bus Selector1/1
  Bus Assignment/1 -> BDB'/1
  BDB_initialize/1 -> Bus Assignment/1
  Bus Selector1/1 -> Bus Assignment/2  "<Qdot_T_opaque>"
  Bus Selector1/13 -> Bus Assignment/14  "<Qdot_C>"
  Bus Selector1/12 -> Bus Assignment/13  "<Qdot_H>"
  Bus Selector1/11 -> Bus Assignment/12  "<Qdot_I_electricity>"
  Bus Selector1/10 -> Bus Assignment/11  "<Qdot_I_light>"
  Bus Selector1/9 -> Bus Assignment/10  "<Qdot_I_person>"
  Bus Selector1/8 -> Bus Assignment/9  "<Qdot_S>"
  Bus Selector1/7 -> Bus Assignment/8  "<Qdot_V_infiltration>"
  Bus Selector1/6 -> Bus Assignment/7  "<Qdot_V_window>"
  Bus Selector1/5 -> Bus Assignment/6  "<Qdot_V_mech>"
  Bus Selector1/4 -> Bus Assignment/5  "<Qdot_T_window>"
  Bus Selector1/3 -> Bus Assignment/4  "<Qdot_T_neighbour>"
  Bus Selector1/2 -> Bus Assignment/3  "<Qdot_T_ground>"

== system building_PHPP_v1/DATALOGGER/z8 ==
  BDB : Inport
  BDB_initialize : carnotUIBK/room_node/EMPTY/BDB_initialize  SystemSampleTime=-1
  Bus Assignment : BusAssignment  AssignedSignals=Qdot_T_opaque,Qdot_T_ground,Qdot_T_neighbour,Qdot_T_window,Qdot_V_mech,Qdot_V_window,Qdot_V_infiltration,Qdot_S,Qdot_I_person,Qdot_I_light,Qdot_I_electricity,Qdot_H,Qdot_C
  Bus Selector1 : BusSelector  OutputSignals=Qdot_T_opaque,Qdot_T_ground,Qdot_T_neighbour,Qdot_T_window,Qdot_V_mech,Qdot_V_window,Qdot_V_infiltration,Qdot_S,Qdot_I_person,Qdot_I_light,Qdot_I_electricity,Qdot_H,Qdot_C
  BDB' : Outport
  wires:
  Bus Selector1/2 -> Bus Assignment/3  "<Qdot_T_ground>"
  Bus Selector1/3 -> Bus Assignment/4  "<Qdot_T_neighbour>"
  Bus Selector1/4 -> Bus Assignment/5  "<Qdot_T_window>"
  Bus Selector1/5 -> Bus Assignment/6  "<Qdot_V_mech>"
  Bus Selector1/6 -> Bus Assignment/7  "<Qdot_V_window>"
  Bus Selector1/7 -> Bus Assignment/8  "<Qdot_V_infiltration>"
  Bus Selector1/8 -> Bus Assignment/9  "<Qdot_S>"
  Bus Selector1/9 -> Bus Assignment/10  "<Qdot_I_person>"
  Bus Selector1/10 -> Bus Assignment/11  "<Qdot_I_light>"
  Bus Selector1/11 -> Bus Assignment/12  "<Qdot_I_electricity>"
  Bus Selector1/12 -> Bus Assignment/13  "<Qdot_H>"
  Bus Selector1/13 -> Bus Assignment/14  "<Qdot_C>"
  Bus Selector1/1 -> Bus Assignment/2  "<Qdot_T_opaque>"
  BDB_initialize/1 -> Bus Assignment/1
  Bus Assignment/1 -> BDB'/1
  BDB/1 -> Bus Selector1/1
